simulink model "PartA1"  (R2019b)
settings: Solver=VariableStepAuto  StartTime=0.0  StopTime=10.0  RelTol=1e-3
settings Model: Creator=visha  LastModifiedBy=visha
settings OptimizationCC: DefaultParameterBehavior=Inlined

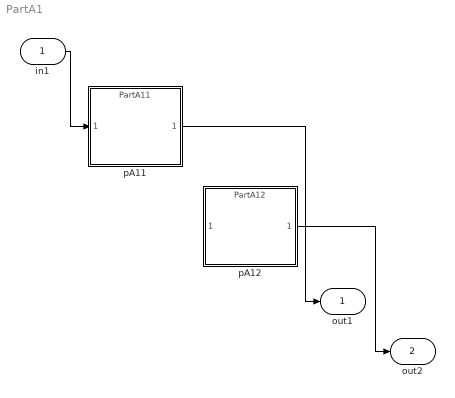
== system PartA1 ==
  in1 : Inport  OutDataTypeStr=double
  pA11 : ModelReference  ModelNameDialog=PartA11  SimulationMode=Normal  ModelReferenceVersion=1.1
  pA12 : ModelReference  ModelNameDialog=PartA12  SimulationMode=Normal  ModelReferenceVersion=1.1
  out1 : Outport  OutDataTypeStr=double
  out2 : Outport  Port=2  OutDataTypeStr=double
  wires:
  in1/1 -> pA11/1
  pA11/1 -> out1/1
  pA12/1 -> out2/1
